simulink model "nid_depth"  (Simulink 7.6)
settings: Solver=FixedStepDiscrete  StartTime=0.0  StopTime=inf  RelTol=1e-3
libraries: nid_lib x2
settings Model: Creator=tchikama  LastModifiedBy=tchikama
settings DataIOCC: SaveOutput=off
settings OptimizationCC: SimCompilerOptimization=On
settings HardwareCC: ProdIntDivRoundTo=Zero  ProdEndianess=LittleEndian  ProdHWDeviceType=Generic->32-bit x86 compatible
settings RTWCC: ProcessScript=grt_make_rtw_hook  RTWCompilerOptimization=On
settings CodeAppCC: MaxIdLength=95

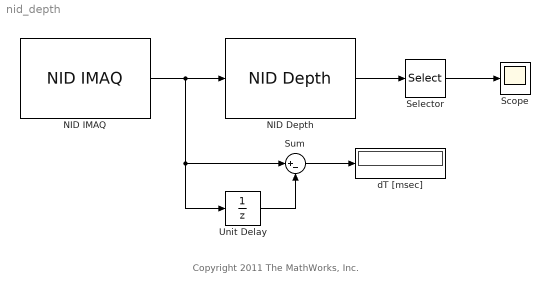
== system nid_depth ==
  note: Copyright 2011 The MathWorks, Inc.
  NID Depth : nid_lib/NID Depth  depthOutput=Depth  viewer=off
  NID IMAQ : nid_lib/NID IMAQ  imaq_depth=on  imaq_motion=off  imaq_image=off  view_point=off  imaq_skeleton=off  imaq_ir=off  mirror_image=off  imaq_sample_time=1/30
  Scope : Scope
      settings: TimeRange=10  YMin=0  SaveName=ScopeData2
  Selector : Selector  NumberOfDimensions=2  IndexOptions=Index vector (dialog),Index vector (dialog)  Indices=480/2,640/2  OutputSizes=1,1
  Sum : Sum  Inputs=|+-
  Unit Delay : UnitDelay  SampleTime=-1
  dT [msec] : Display
  wires:
  NID Depth/1 -> Selector/1
  NID IMAQ/1 -> Unit Delay/1, Sum/1, NID Depth/1
  Unit Delay/1 -> Sum/2
  Sum/1 -> dT [msec]/1
  Selector/1 -> Scope/1
